simulink model "DYN_01x"  (R2018b)
(part 6 of 13)

a2*de1*m6*x6*cos(e2)^2*cos(e3)*cos(e6)*sin(e4) - a3*de1*m6*x6*cos(e2)^2*cos(e4)*cos(e5)*sin(e6) - a3*de1*m6*x6*cos(e3)^2*cos(e4)*cos(e5)*sin(e6) + 2*I6xy*de1*cos(e2)*cos(e3)*cos(e4)^2*cos(e5)^2*sin(e2)*sin(e3) - 4*I6xy*de1*cos(e2)*cos(e3)*cos(e4)^2*cos(e6)^2*sin(e2)*sin(e3) - 4*I6xy*de1*cos(e2)*cos(e3)*cos(e5)^2*cos(e6)^2*sin(e2)*sin(e3) - 4*I6zx*de1*cos(e2)*cos(e3)^2*cos(e4)*cos(e5)^2*sin(e2)*sin(e6) - 4*I6zx*de1*cos(e2)^2*cos(e3)*cos(e4)*cos(e5)^2*sin(e3)*sin(e6) - 2*I6zx*de1*cos(e2)^2*cos(e3)^2*cos(e4)*cos(e6)*sin(e4)*sin(e5) - a2*de1*m6*y6*cos(e2)^2*cos(e3)*sin(e4)*sin(e6) - a2*de1*m6*y6*cos(e2)^2*cos(e6)*sin(e3)*sin(e5) + 4*I6xx*de1*cos(e2)*cos(e3)^2*cos(e6)^2*sin(e2)*sin(e4)*sin(e5) + 4*I6xx*de1*cos(e2)^2*cos(e3)*cos(e6)^2*sin(e3)*sin(e4)*sin(e5) + 2*I6xy*de2*cos(e4)*cos(e5)^2*cos(e6)^2*sin(e2)*sin(e3)*sin(e4) + 2*I6xy*de3*cos(e4)*cos(e5)^2*cos(e6)^2*sin(e2)*sin(e3)*sin(e4) - 4*I6yy*de1*cos(e2)*cos(e3)^2*cos(e6)^2*sin(e2)*sin(e4)*sin(e5) - 4*I6yy*de1*cos(e2)^2*cos(e3)*cos(e6)^2*sin(e3)*sin(e4)*sin(e5) + 2*I6yz*de1*cos(e2)^2*cos(e3)^2*cos(e4)*sin(e4)*sin(e5)*sin(e6) + 2*de2*m6*x6^2*cos(e2)*cos(e3)*cos(e4)^2*cos(e5)*cos(e6)^2 + 2*de3*m6*x6^2*cos(e2)*cos(e3)*cos(e4)^2*cos(e5)*cos(e6)^2 - 2*de2*m6*y6^2*cos(e2)*cos(e3)*cos(e4)^2*cos(e5)*cos(e6)^2 - 2*de3*m6*y6^2*cos(e2)*cos(e3)*cos(e4)^2*cos(e5)*cos(e6)^2 - 2*de5*m6*x6*y6*cos(e2)*cos(e3)*cos(e6)^2*sin(e4) + de1*m6*y6*z6*cos(e2)^2*cos(e5)*cos(e6)*sin(e5) + de1*m6*y6*z6*cos(e3)^2*cos(e5)*cos(e6)*sin(e5) - de1*m6*y6*z6*cos(e4)^2*cos(e5)*cos(e6)*sin(e5) - a2*de1*m6*x6*cos(e2)^2*sin(e3)*sin(e5)*sin(e6) - 2*de1*m6*x6^2*cos(e2)^2*cos(e3)^2*cos(e4)*cos(e5)*sin(e4) - 2*de1*m6*x6^2*cos(e2)^2*cos(e4)*cos(e5)*cos(e6)^2*sin(e4) - 2*de1*m6*x6^2*cos(e3)^2*cos(e4)*cos(e5)*cos(e6)^2*sin(e4) - 2*de1*m6*x6*y6*cos(e2)^2*cos(e3)^2*cos(e4)^2*cos(e5)^2 + 4*de1*m6*x6*y6*cos(e2)^2*cos(e3)^2*cos(e4)^2*cos(e6)^2 + 4*de1*m6*x6*y6*cos(e2)^2*cos(e3)^2*cos(e5)^2*cos(e6)^2 - 2*de1*m6*x6*y6*cos(e2)^2*cos(e4)^2*cos(e5)^2*cos(e6)^2 - 2*de1*m6*x6*y6*cos(e3)^2*cos(e4)^2*cos(e5)^2*cos(e6)^2 + 2*de1*m6*y6^2*cos(e2)^2*cos(e3)^2*cos(e4)*cos(e5)*sin(e4) + 2*de1*m6*y6^2*cos(e2)^2*cos(e4)*cos(e5)*cos(e6)^2*sin(e4) + 2*de1*m6*y6^2*cos(e3)^2*cos(e4)*cos(e5)*cos(e6)^2*sin(e4) + de1*m6*x6*z6*cos(e2)^2*cos(e5)*sin(e5)*sin(e6) + de1*m6*x6*z6*cos(e3)^2*cos(e5)*sin(e5)*sin(e6) - de1*m6*x6*z6*cos(e4)^2*cos(e5)*sin(e5)*sin(e6) - 2*I6xy*de5*cos(e2)*cos(e3)*cos(e4)*cos(e5)*cos(e6)*sin(e6) - 2*de2*m6*x6^2*cos(e4)^2*cos(e5)*cos(e6)^2*sin(e2)*sin(e3) - 2*de3*m6*x6^2*cos(e4)^2*cos(e5)*cos(e6)^2*sin(e2)*sin(e3) + 2*de2*m6*y6^2*cos(e4)^2*cos(e5)*cos(e6)^2*sin(e2)*sin(e3) + 2*de3*m6*y6^2*cos(e4)^2*cos(e5)*cos(e6)^2*sin(e2)*sin(e3) + 2*de5*m6*x6*y6*cos(e6)^2*sin(e2)*sin(e3)*sin(e4) + I6xx*de2*cos(e2)*cos(e3)*cos(e4)*cos(e6)*sin(e4)*sin(e6) + I6xx*de3*cos(e2)*cos(e3)*cos(e4)*cos(e6)*sin(e4)*sin(e6) - I6yy*de2*cos(e2)*cos(e3)*cos(e4)*cos(e6)*sin(e4)*sin(e6) - I6yy*de3*cos(e2)*cos(e3)*cos(e4)*cos(e6)*sin(e4)*sin(e6) - 4*I6xx*de1*cos(e2)^2*cos(e3)^2*cos(e4)*cos(e5)*cos(e6)^2*sin(e4) + 4*I6yy*de1*cos(e2)^2*cos(e3)^2*cos(e4)*cos(e5)*cos(e6)^2*sin(e4) - 2*I6yz*de1*cos(e2)^2*cos(e3)^2*cos(e4)^2*cos(e5)*cos(e6)*sin(e5) - 4*I6xx*de1*cos(e2)*cos(e3)*cos(e6)*sin(e2)*sin(e3)*sin(e6) + 2*I6xy*de2*cos(e2)*cos(e4)*cos(e6)*sin(e3)*sin(e5)*sin(e6) + 2*I6xy*de2*cos(e3)*cos(e4)*cos(e6)*sin(e2)*sin(e5)*sin(e6) + 2*I6xy*de3*cos(e2)*cos(e4)*cos(e6)*sin(e3)*sin(e5)*sin(e6) + 2*I6xy*de3*cos(e3)*cos(e4)*cos(e6)*sin(e2)*sin(e5)*sin(e6) - 2*I6xy*de4*cos(e2)*cos(e3)*cos(e6)*sin(e4)*sin(e5)*sin(e6) + 2*I6xy*de5*cos(e4)*cos(e5)*cos(e6)*sin(e2)*sin(e3)*sin(e6) + 4*I6yy*de1*cos(e2)*cos(e3)*cos(e6)*sin(e2)*sin(e3)*sin(e6) + 2*a3*de1*m6*x6*cos(e2)^2*cos(e3)^2*cos(e6)*sin(e4) - 2*I6zx*de1*cos(e2)^2*cos(e3)^2*cos(e4)^2*cos(e5)*sin(e5)*sin(e6) - 2*d4*de1*m6*y6*cos(e2)^2*cos(e3)^2*cos(e6)*sin(e5) - I6xx*de2*cos(e4)*cos(e6)*sin(e2)*sin(e3)*sin(e4)*sin(e6) - 4*I6xy*de1*cos(e2)*cos(e6)*sin(e2)*sin(e4)*sin(e5)*sin(e6) - I6xx*de3*cos(e4)*cos(e6)*sin(e2)*sin(e3)*sin(e4)*sin(e6) - 4*I6xy*de1*cos(e3)*cos(e6)*sin(e3)*sin(e4)*sin(e5)*sin(e6) + I6yy*de2*cos(e4)*cos(e6)*sin(e2)*sin(e3)*sin(e4)*sin(e6) + I6yy*de3*cos(e4)*cos(e6)*sin(e2)*sin(e3)*sin(e4)*sin(e6) - a1*de1*m6*y6*cos(e2)*cos(e4)*cos(e5)*cos(e6)*sin(e3) - a1*de1*m6*y6*cos(e3)*cos(e4)*cos(e5)*cos(e6)*sin(e2) + a3*de4*m6*y6*cos(e2)*cos(e4)*cos(e5)*cos(e6)*sin(e3) + a3*de4*m6*y6*cos(e3)*cos(e4)*cos(e5)*cos(e6)*sin(e2) + d4*de4*m6*x6*cos(e2)*cos(e3)*cos(e4)*cos(e5)*sin(e6) + d4*de6*m6*x6*cos(e2)*cos(e3)*cos(e5)*cos(e6)*sin(e4) + I6xx*de2*cos(e2)*cos(e3)*cos(e4)*cos(e5)^2*cos(e6)*sin(e4)*sin(e6) + I6xx*de3*cos(e2)*cos(e3)*cos(e4)*cos(e5)^2*cos(e6)*sin(e4)*sin(e6) - I6yy*de2*cos(e2)*cos(e3)*cos(e4)*cos(e5)^2*cos(e6)*sin(e4)*sin(e6) - I6yy*de3*cos(e2)*cos(e3)*cos(e4)*cos(e5)^2*cos(e6)*sin(e4)*sin(e6) + d4*de1*m6*y6*cos(e2)*cos(e4)*cos(e5)*cos(e6)*sin(e2) + d4*de1*m6*y6*cos(e3)*cos(e4)*cos(e5)*cos(e6)*sin(e3) + de6*m6*y6*z6*cos(e2)*cos(e3)*cos(e4)*cos(e5)*cos(e6) - a1*de1*m6*x6*cos(e2)*cos(e4)*cos(e5)*sin(e3)*sin(e6) - a1*de1*m6*x6*cos(e3)*cos(e4)*cos(e5)*sin(e2)*sin(e6) + a3*de4*m6*x6*cos(e2)*cos(e4)*cos(e5)*sin(e3)*sin(e6) + a3*de4*m6*x6*cos(e3)*cos(e4)*cos(e5)*sin(e2)*sin(e6) + a3*de6*m6*x6*cos(e2)*cos(e5)*cos(e6)*sin(e3)*sin(e4) + a3*de6*m6*x6*cos(e3)*cos(e5)*cos(e6)*sin(e2)*sin(e4) - a2*de1*m6*y6*cos(e2)*cos(e3)*cos(e6)*sin(e2)*sin(e5) + d4*de1*m6*x6*cos(e2)*cos(e4)*cos(e5)*sin(e2)*sin(e6) + d4*de1*m6*x6*cos(e3)*cos(e4)*cos(e5)*sin(e3)*sin(e6) + 2*I6xx*de1*cos(e2)*cos(e3)*cos(e4)^2*cos(e6)*sin(e2)*sin(e3)*sin(e6) + 2*I6xx*de1*cos(e2)*cos(e3)*cos(e5)^2*cos(e6)*sin(e2)*sin(e3)*sin(e6) - 2*I6yy*de1*cos(e2)*cos(e3)*cos(e4)^2*cos(e6)*sin(e2)*sin(e3)*sin(e6) - 2*I6yy*de1*cos(e2)*cos(e3)*cos(e5)^2*cos(e6)*sin(e2)*sin(e3)*sin(e6) - d4*de4*m6*y6*cos(e4)*cos(e5)*cos(e6)*sin(e2)*sin(e3) - d4*de5*m6*y6*cos(e2)*cos(e3)*cos(e6)*sin(e4)*sin(e5) - d4*de6*m6*y6*cos(e2)*cos(e3)*cos(e5)*sin(e4)*sin(e6) - de4*m6*x6*y6*cos(e2)*cos(e3)*cos(e4)*cos(e5)*sin(e5) + 2*de2*m6*x6*y6*cos(e2)*cos(e3)*cos(e5)*cos(e6)*sin(e6) + 2*de3*m6*x6*y6*cos(e2)*cos(e3)*cos(e5)*cos(e6)*sin(e6) + de4*m6*x6*z6*cos(e2)*cos(e3)*cos(e5)*cos(e6)*sin(e4) + de6*m6*x6*z6*cos(e2)*cos(e3)*cos(e4)*cos(e5)*sin(e6) - a2*de1*m6*x6*cos(e2)*cos(e6)*sin(e2)*sin(e3)*sin(e4) - a2*de1*m6*x6*cos(e2)*cos(e3)*sin(e2)*sin(e5)*sin(e6) - a3*de5*m6*y6*cos(e2)*cos(e6)*sin(e3)*sin(e4)*sin(e5) - a3*de5*m6*y6*cos(e3)*cos(e6)*sin(e2)*sin(e4)*sin(e5) - a3*de6*m6*y6*cos(e2)*cos(e5)*sin(e3)*sin(e4)*sin(e6) - a3*de6*m6*y6*cos(e3)*cos(e5)*sin(e2)*sin(e4)*sin(e6) - d4*de4*m6*x6*cos(e4)*cos(e5)*sin(e2)*sin(e3)*sin(e6) - d4*de5*m6*x6*cos(e2)*cos(e3)*sin(e4)*sin(e5)*sin(e6) - d4*de6*m6*x6*cos(e5)*cos(e6)*sin(e2)*sin(e3)*sin(e4) + 8*I6xy*de1*cos(e2)*cos(e3)^2*cos(e6)*sin(e2)*sin(e4)*sin(e5)*sin(e6) + 8*I6xy*de1*cos(e2)^2*cos(e3)*cos(e6)*sin(e3)*sin(e4)*sin(e5)*sin(e6) - I6xx*de2*cos(e4)*cos(e5)^2*cos(e6)*sin(e2)*sin(e3)*sin(e4)*sin(e6) - I6xx*de3*cos(e4)*cos(e5)^2*cos(e6)*sin(e2)*sin(e3)*sin(e4)*sin(e6) + I6yy*de2*cos(e4)*cos(e5)^2*cos(e6)*sin(e2)*sin(e3)*sin(e4)*sin(e6) + I6yy*de3*cos(e4)*cos(e5)^2*cos(e6)*sin(e2)*sin(e3)*sin(e4)*sin(e6) - 2*de1*m6*x6*y6*cos(e2)*cos(e4)*cos(e5)*sin(e2)*sin(e5) - 2*de1*m6*x6*y6*cos(e3)*cos(e4)*cos(e5)*sin(e3)*sin(e5) - 4*de1*m6*x6*y6*cos(e4)*cos(e5)*cos(e6)*sin(e4)*sin(e6) + de1*m6*x6*z6*cos(e2)*cos(e5)*cos(e6)*sin(e2)*sin(e4) + de1*m6*x6*z6*cos(e3)*cos(e5)*cos(e6)*sin(e3)*sin(e4) - de4*m6*y6*z6*cos(e2)*cos(e3)*cos(e5)*sin(e4)*sin(e6) - de4*m6*y6*z6*cos(e2)*cos(e5)*cos(e6)*sin(e3)*sin(e5) - de4*m6*y6*z6*cos(e3)*cos(e5)*cos(e6)*sin(e2)*sin(e5) - de6*m6*y6*z6*cos(e4)*cos(e5)*cos(e6)*sin(e2)*sin(e3) - a3*de5*m6*x6*cos(e2)*sin(e3)*sin(e4)*sin(e5)*sin(e6) - a3*de5*m6*x6*cos(e3)*sin(e2)*sin(e4)*sin(e5)*sin(e6) + a2*de1*m6*y6*cos(e2)*sin(e2)*sin(e3)*sin(e4)*sin(e6) + d4*de5*m6*y6*cos(e6)*sin(e2)*sin(e3)*sin(e4)*sin(e5) + d4*de6*m6*y6*cos(e5)*sin(e2)*sin(e3)*sin(e4)*sin(e6) - de2*m6*x6*y6*cos(e2)*cos(e5)*sin(e3)*sin(e4)*sin(e5) - de2*m6*x6*y6*cos(e3)*cos(e5)*sin(e2)*sin(e4)*sin(e5) - de3*m6*x6*y6*cos(e2)*cos(e5)*sin(e3)*sin(e4)*sin(e5) - de3*m6*x6*y6*cos(e3)*cos(e5)*sin(e2)*sin(e4)*sin(e5) + de4*m6*x6*y6*cos(e4)*cos(e5)*sin(e2)*sin(e3)*sin(e5) - 2*de2*m6*x6*y6*cos(e5)*cos(e6)*sin(e2)*sin(e3)*sin(e6) - 2*de3*m6*x6*y6*cos(e5)*cos(e6)*sin(e2)*sin(e3)*sin(e6) + 2*de5*m6*x6*y6*cos(e2)*cos(e6)*sin(e3)*sin(e5)*sin(e6) + 2*de5*m6*x6*y6*cos(e3)*cos(e6)*sin(e2)*sin(e5)*sin(e6) - de4*m6*x6*z6*cos(e5)*cos(e6)*sin(e2)*sin(e3)*sin(e4) - de4*m6*x6*z6*cos(e2)*cos(e5)*sin(e3)*sin(e5)*sin(e6) - de4*m6*x6*z6*cos(e3)*cos(e5)*sin(e2)*sin(e5)*sin(e6) - de6*m6*x6*z6*cos(e4)*cos(e5)*sin(e2)*sin(e3)*sin(e6) - de1*m6*y6*z6*cos(e2)*cos(e5)*sin(e2)*sin(e4)*sin(e6) - de1*m6*y6*z6*cos(e3)*cos(e5)*sin(e3)*sin(e4)*sin(e6) + d4*de5*m6*x6*sin(e2)*sin(e3)*sin(e4)*sin(e5)*sin(e6) + 2*de1*m6*x6^2*cos(e2)^2*cos(e3)^2*cos(e4)^2*cos(e5)^2*cos(e6)*sin(e6) - 2*de1*m6*y6^2*cos(e2)^2*cos(e3)^2*cos(e4)^2*cos(e5)^2*cos(e6)*sin(e6) + de4*m6*y6*z6*cos(e5)*sin(e2)*sin(e3)*sin(e4)*sin(e6) + a2*de1*m6*y6*cos(e2)^2*cos(e3)*cos(e4)*cos(e5)*cos(e6) + a2*de1*m6*x6*cos(e2)^2*cos(e3)*cos(e4)*cos(e5)*sin(e6) - 8*I6xy*de1*cos(e2)*cos(e3)^2*cos(e4)*cos(e5)*cos(e6)^2*sin(e2)*sin(e5) - 8*I6xy*de1*cos(e2)^2*cos(e3)*cos(e4)*cos(e5)*cos(e6)^2*sin(e3)*sin(e5) - 8*I6xy*de1*cos(e2)^2*cos(e3)^2*cos(e4)*cos(e5)*cos(e6)*sin(e4)*sin(e6) + de4*m6*y6*z6*cos(e2)*cos(e3)*cos(e4)*cos(e5)^2*cos(e6) - 2*a3*de1*m6*y6*cos(e2)*cos(e3)^2*cos(e6)*sin(e2)*sin(e5) - 2*a3*de1*m6*y6*cos(e2)^2*cos(e3)*cos(e6)*sin(e3)*sin(e5) - 2*d4*de1*m6*x6*cos(e2)*cos(e3)^2*cos(e6)*sin(e2)*sin(e4) - 2*d4*de1*m6*x6*cos(e2)^2*cos(e3)*cos(e6)*sin(e3)*sin(e4) + de2*m6*x6*y6*cos(e2)*cos(e3)*cos(e4)*cos(e5)^2*sin(e4) - 2*de2*m6*x6*y6*cos(e2)*cos(e3)*cos(e4)*cos(e6)^2*sin(e4) + de3*m6*x6*y6*cos(e2)*cos(e3)*cos(e4)*cos(e5)^2*sin(e4) - 2*de3*m6*x6*y6*cos(e2)*cos(e3)*cos(e4)*cos(e6)^2*sin(e4) - de2*m6*x6*z6*cos(e2)*cos(e3)*cos(e4)^2*cos(e6)*sin(e5) - de3*m6*x6*z6*cos(e2)*cos(e3)*cos(e4)^2*cos(e6)*sin(e5) + de4*m6*x6*z6*cos(e2)*cos(e3)*cos(e4)*cos(e5)^2*sin(e6) + 2*de1*m6*y6*z6*cos(e2)*cos(e3)^2*cos(e4)*cos(e6)*sin(e2) + 2*de1*m6*y6*z6*cos(e2)^2*cos(e3)*cos(e4)*cos(e6)*sin(e3) + 2*de1*m6*y6*z6*cos(e2)*cos(e4)*cos(e5)^2*cos(e6)*sin(e2) + 2*de1*m6*y6*z6*cos(e3)*cos(e4)*cos(e5)^2*cos(e6)*sin(e3) - 2*a3*de1*m6*x6*cos(e2)*cos(e3)^2*sin(e2)*sin(e5)*sin(e6) - 2*a3*de1*m6*x6*cos(e2)^2*cos(e3)*sin(e3)*sin(e5)*sin(e6) + 2*d4*de1*m6*y6*cos(e2)*cos(e3)^2*sin(e2)*sin(e4)*sin(e6) + 2*d4*de1*m6*y6*cos(e2)^2*cos(e3)*sin(e3)*sin(e4)*sin(e6) + 2*de1*m6*x6*y6*cos(e2)*cos(e3)*cos(e4)^2*sin(e2)*sin(e3) + 2*de1*m6*x6*y6*cos(e2)*cos(e3)*cos(e5)^2*sin(e2)*sin(e3) + 8*de1*m6*x6*y6*cos(e2)*cos(e3)*cos(e6)^2*sin(e2)*sin(e3) + 2*de1*m6*x6*z6*cos(e2)*cos(e3)^2*cos(e4)*sin(e2)*sin(e6) + 2*de1*m6*x6*z6*cos(e2)^2*cos(e3)*cos(e4)*sin(e3)*sin(e6) + 2*de1*m6*x6*z6*cos(e2)*cos(e4)*cos(e5)^2*sin(e2)*sin(e6) + 2*de1*m6*x6*z6*cos(e3)*cos(e4)*cos(e5)^2*sin(e3)*sin(e6) + de1*m6*x6*z6*cos(e2)^2*cos(e4)*cos(e6)*sin(e4)*sin(e5) + de1*m6*x6*z6*cos(e3)^2*cos(e4)*cos(e6)*sin(e4)*sin(e5) + de2*m6*y6*z6*cos(e2)*cos(e3)*cos(e4)^2*sin(e5)*sin(e6) + de2*m6*y6*z6*cos(e2)*cos(e5)^2*cos(e6)*sin(e3)*sin(e4) + de2*m6*y6*z6*cos(e3)*cos(e5)^2*cos(e6)*sin(e2)*sin(e4) + de3*m6*y6*z6*cos(e2)*cos(e3)*cos(e4)^2*sin(e5)*sin(e6) + de3*m6*y6*z6*cos(e2)*cos(e5)^2*cos(e6)*sin(e3)*sin(e4) + de3*m6*y6*z6*cos(e3)*cos(e5)^2*cos(e6)*sin(e2)*sin(e4) - de4*m6*y6*z6*cos(e4)*cos(e5)^2*cos(e6)*sin(e2)*sin(e3) - de2*m6*x6*y6*cos(e4)*cos(e5)^2*sin(e2)*sin(e3)*sin(e4) + 2*de2*m6*x6*y6*cos(e4)*cos(e6)^2*sin(e2)*sin(e3)*sin(e4) - de3*m6*x6*y6*cos(e4)*cos(e5)^2*sin(e2)*sin(e3)*sin(e4) + 2*de3*m6*x6*y6*cos(e4)*cos(e6)^2*sin(e2)*sin(e3)*sin(e4) + de2*m6*x6*z6*cos(e2)*cos(e5)^2*sin(e3)*sin(e4)*sin(e6) + de2*m6*x6*z6*cos(e3)*cos(e5)^2*sin(e2)*sin(e4)*sin(e6) + de2*m6*x6*z6*cos(e4)^2*cos(e6)*sin(e2)*sin(e3)*sin(e5) + de3*m6*x6*z6*cos(e2)*cos(e5)^2*sin(e3)*sin(e4)*sin(e6) + de3*m6*x6*z6*cos(e3)*cos(e5)^2*sin(e2)*sin(e4)*sin(e6) + de3*m6*x6*z6*cos(e4)^2*cos(e6)*sin(e2)*sin(e3)*sin(e5) - de4*m6*x6*z6*cos(e4)*cos(e5)^2*sin(e2)*sin(e3)*sin(e6) - de1*m6*y6*z6*cos(e2)^2*cos(e4)*sin(e4)*sin(e5)*sin(e6) - de1*m6*y6*z6*cos(e3)^2*cos(e4)*sin(e4)*sin(e5)*sin(e6) - I6xx*de4*cos(e2)*cos(e3)*cos(e4)*cos(e5)*cos(e6)*sin(e5)*sin(e6) + I6yz*de2*cos(e2)*cos(e3)*cos(e4)*cos(e5)*cos(e6)*sin(e4)*sin(e5) + I6yz*de3*cos(e2)*cos(e3)*cos(e4)*cos(e5)*cos(e6)*sin(e4)*sin(e5) + I6yy*de4*cos(e2)*cos(e3)*cos(e4)*cos(e5)*cos(e6)*sin(e5)*sin(e6) - 4*de1*m6*x6^2*cos(e2)*cos(e3)^2*cos(e6)^2*sin(e2)*sin(e4)*sin(e5) - 4*de1*m6*x6^2*cos(e2)^2*cos(e3)*cos(e6)^2*sin(e3)*sin(e4)*sin(e5) + 4*de1*m6*y6^2*cos(e2)*cos(e3)^2*cos(e6)^2*sin(e2)*sin(e4)*sin(e5) + 4*de1*m6*y6^2*cos(e2)^2*cos(e3)*cos(e6)^2*sin(e3)*sin(e4)*sin(e5) - de2*m6*y6*z6*cos(e4)^2*sin(e2)*sin(e3)*sin(e5)*sin(e6) - de3*m6*y6*z6*cos(e4)^2*sin(e2)*sin(e3)*sin(e5)*sin(e6) + 2*a3*de1*m6*y6*cos(e2)^2*cos(e3)^2*cos(e4)*cos(e5)*cos(e6) - 2*I6xx*de1*cos(e2)*cos(e3)*cos(e4)*cos(e5)*sin(e2)*sin(e3)*sin(e4) - 2*I6xx*de1*cos(e2)*cos(e4)*cos(e5)*cos(e6)*sin(e2)*sin(e5)*sin(e6) - 2*I6xx*de1*cos(e3)*cos(e4)*cos(e5)*cos(e6)*sin(e3)*sin(e5)*sin(e6) + 2*I6yy*de1*cos(e2)*cos(e3)*cos(e4)*cos(e5)*sin(e2)*sin(e3)*sin(e4) + 2*I6yz*de1*cos(e2)*cos(e3)*cos(e5)*cos(e6)*sin(e2)*sin(e3)*sin(e5) + 2*I6yy*de1*cos(e2)*cos(e4)*cos(e5)*cos(e6)*sin(e2)*sin(e5)*sin(e6) + 2*I6yy*de1*cos(e3)*cos(e4)*cos(e5)*cos(e6)*sin(e3)*sin(e5)*sin(e6) + I6zx*de2*cos(e2)*cos(e3)*cos(e4)*cos(e5)*sin(e4)*sin(e5)*sin(e6) + I6zx*de3*cos(e2)*cos(e3)*cos(e4)*cos(e5)*sin(e4)*sin(e5)*sin(e6) + 2*a3*de1*m6*x6*cos(e2)^2*cos(e3)^2*cos(e4)*cos(e5)*sin(e6) - 4*I6xy*de1*cos(e2)*cos(e3)*cos(e4)^2*cos(e5)^2*cos(e6)^2*sin(e2)*sin(e3) - I6xx*de2*cos(e2)*cos(e5)*cos(e6)*sin(e3)*sin(e4)*sin(e5)*sin(e6) - I6xx*de2*cos(e3)*cos(e5)*cos(e6)*sin(e2)*sin(e4)*sin(e5)*sin(e6) - I6xx*de3*cos(e2)*cos(e5)*cos(e6)*sin(e3)*sin(e4)*sin(e5)*sin(e6) - I6xx*de3*cos(e3)*cos(e5)*cos(e6)*sin(e2)*sin(e4)*sin(e5)*sin(e6) + I6xx*de4*cos(e4)*cos(e5)*cos(e6)*sin(e2)*sin(e3)*sin(e5)*sin(e6) - I6yz*de2*cos(e4)*cos(e5)*cos(e6)*sin(e2)*sin(e3)*sin(e4)*sin(e5) + I6yy*de2*cos(e2)*cos(e5)*cos(e6)*sin(e3)*sin(e4)*sin(e5)*sin(e6) + I6yy*de2*cos(e3)*cos(e5)*cos(e6)*sin(e2)*sin(e4)*sin(e5)*sin(e6) - I6yz*de3*cos(e4)*cos(e5)*cos(e6)*sin(e2)*sin(e3)*sin(e4)*sin(e5) + I6yy*de3*cos(e2)*cos(e5)*cos(e6)*sin(e3)*sin(e4)*sin(e5)*sin(e6) + I6yy*de3*cos(e3)*cos(e5)*cos(e6)*sin(e2)*sin(e4)*sin(e5)*sin(e6) - I6yy*de4*cos(e4)*cos(e5)*cos(e6)*sin(e2)*sin(e3)*sin(e5)*sin(e6) + 2*I6zx*de1*cos(e2)*cos(e3)*cos(e5)*sin(e2)*sin(e3)*sin(e5)*sin(e6) - I6zx*de2*cos(e4)*cos(e5)*sin(e2)*sin(e3)*sin(e4)*sin(e5)*sin(e6) - I6zx*de3*cos(e4)*cos(e5)*sin(e2)*sin(e3)*sin(e4)*sin(e5)*sin(e6) - de2*m6*x6^2*cos(e2)*cos(e3)*cos(e4)*cos(e6)*sin(e4)*sin(e6) - de3*m6*x6^2*cos(e2)*cos(e3)*cos(e4)*cos(e6)*sin(e4)*sin(e6) + de2*m6*y6^2*cos(e2)*cos(e3)*cos(e4)*cos(e6)*sin(e4)*sin(e6) + de3*m6*y6^2*cos(e2)*cos(e3)*cos(e4)*cos(e6)*sin(e4)*sin(e6) - 2*de1*m6*y6*z6*cos(e2)^2*cos(e3)^2*cos(e5)*cos(e6)*sin(e5) + de1*m6*y6*z6*cos(e2)^2*cos(e4)^2*cos(e5)*cos(e6)*sin(e5) + de1*m6*y6*z6*cos(e3)^2*cos(e4)^2*cos(e5)*cos(e6)*sin(e5) + 4*de1*m6*x6^2*cos(e2)^2*cos(e3)^2*cos(e4)*cos(e5)*cos(e6)^2*sin(e4) + 4*de1*m6*x6*y6*cos(e2)^2*cos(e3)^2*cos(e4)^2*cos(e5)^2*cos(e6)^2 - 4*de1*m6*y6^2*cos(e2)^2*cos(e3)^2*cos(e4)*cos(e5)*cos(e6)^2*sin(e4) + 4*de1*m6*x6^2*cos(e2)*cos(e3)*cos(e6)*sin(e2)*sin(e3)*sin(e6) - 4*de1*m6*y6^2*cos(e2)*cos(e3)*cos(e6)*sin(e2)*sin(e3)*sin(e6) - 2*de1*m6*x6*z6*cos(e2)^2*cos(e3)^2*cos(e5)*sin(e5)*sin(e6) + de1*m6*x6*z6*cos(e2)^2*cos(e4)^2*cos(e5)*sin(e5)*sin(e6) + de1*m6*x6*z6*cos(e3)^2*cos(e4)^2*cos(e5)*sin(e5)*sin(e6) + d4*de4*m6*y6*cos(e2)*cos(e3)*cos(e4)*cos(e5)*cos(e6) + de2*m6*x6^2*cos(e4)*cos(e6)*sin(e2)*sin(e3)*sin(e4)*sin(e6) + de3*m6*x6^2*cos(e4)*cos(e6)*sin(e2)*sin(e3)*sin(e4)*sin(e6) - de2*m6*y6^2*cos(e4)*cos(e6)*sin(e2)*sin(e3)*sin(e4)*sin(e6) - de3*m6*y6^2*cos(e4)*cos(e6)*sin(e2)*sin(e3)*sin(e4)*sin(e6) - de2*m6*x6^2*cos(e2)*cos(e3)*cos(e4)*cos(e5)^2*cos(e6)*sin(e4)*sin(e6) - de3*m6*x6^2*cos(e2)*cos(e3)*cos(e4)*cos(e5)^2*cos(e6)*sin(e4)*sin(e6) + de2*m6*y6^2*cos(e2)*cos(e3)*cos(e4)*cos(e5)^2*cos(e6)*sin(e4)*sin(e6) + de3*m6*y6^2*cos(e2)*cos(e3)*cos(e4)*cos(e5)^2*cos(e6)*sin(e4)*sin(e6) + 2*de2*m6*x6*y6*cos(e2)*cos(e4)*cos(e6)*sin(e3)*sin(e5)*sin(e6) + 2*de2*m6*x6*y6*cos(e3)*cos(e4)*cos(e6)*sin(e2)*sin(e5)*sin(e6) + 2*de3*m6*x6*y6*cos(e2)*cos(e4)*cos(e6)*sin(e3)*sin(e5)*sin(e6) + 2*de3*m6*x6*y6*cos(e3)*cos(e4)*cos(e6)*sin(e2)*sin(e5)*sin(e6) - 2*de4*m6*x6*y6*cos(e2)*cos(e3)*cos(e6)*sin(e4)*sin(e5)*sin(e6) + 2*de5*m6*x6*y6*cos(e4)*cos(e5)*cos(e6)*sin(e2)*sin(e3)*sin(e6) - 2*de1*m6*y6*z6*cos(e2)^2*cos(e3)^2*cos(e4)^2*cos(e5)*cos(e6)*sin(e5) - 2*de1*m6*x6^2*cos(e2)*cos(e3)*cos(e4)^2*cos(e6)*sin(e2)*sin(e3)*sin(e6) - 2*de1*m6*x6^2*cos(e2)*cos(e3)*cos(e5)^2*cos(e6)*sin(e2)*sin(e3)*sin(e6) + 2*de1*m6*y6^2*cos(e2)*cos(e3)*cos(e4)^2*cos(e6)*sin(e2)*sin(e3)*sin(e6) + 2*de1*m6*y6^2*cos(e2)*cos(e3)*cos(e5)^2*cos(e6)*sin(e2)*sin(e3)*sin(e6) - 2*de1*m6*x6*z6*cos(e2)^2*cos(e3)^2*cos(e4)^2*cos(e5)*sin(e5)*sin(e6) - 4*de1*m6*x6*y6*cos(e2)*cos(e6)*sin(e2)*sin(e4)*sin(e5)*sin(e6) - 4*de1*m6*x6*y6*cos(e3)*cos(e6)*sin(e3)*sin(e4)*sin(e5)*sin(e6) + de2*m6*x6^2*cos(e4)*cos(e5)^2*cos(e6)*sin(e2)*sin(e3)*sin(e4)*sin(e6) + de3*m6*x6^2*cos(e4)*cos(e5)^2*cos(e6)*sin(e2)*sin(e3)*sin(e4)*sin(e6) - de2*m6*y6^2*cos(e4)*cos(e5)^2*cos(e6)*sin(e2)*sin(e3)*sin(e4)*sin(e6) - de3*m6*y6^2*cos(e4)*cos(e5)^2*cos(e6)*sin(e2)*sin(e3)*sin(e4)*sin(e6) + 2*de4*m6*x6*y6*cos(e6)*sin(e2)*sin(e3)*sin(e4)*sin(e5)*sin(e6) - 2*d4*de1*m6*y6*cos(e2)*cos(e3)^2*cos(e4)*cos(e5)*cos(e6)*sin(e2) - 2*d4*de1*m6*y6*cos(e2)^2*cos(e3)*cos(e4)*cos(e5)*cos(e6)*sin(e3) - 2*d4*de1*m6*x6*cos(e2)*cos(e3)^2*cos(e4)*cos(e5)*sin(e2)*sin(e6) - 2*d4*de1*m6*x6*cos(e2)^2*cos(e3)*cos(e4)*cos(e5)*sin(e3)*sin(e6) + 2*I6xx*de1*cos(e2)*cos(e3)*cos(e4)^2*cos(e5)^2*cos(e6)*sin(e2)*sin(e3)*sin(e6) - 2*I6yy*de1*cos(e2)*cos(e3)*cos(e4)^2*cos(e5)^2*cos(e6)*sin(e2)*sin(e3)*sin(e6) - 4*de2*m6*x6*y6*cos(e2)*cos(e3)*cos(e4)^2*cos(e5)*cos(e6)*sin(e6) - 4*de3*m6*x6*y6*cos(e2)*cos(e3)*cos(e4)^2*cos(e5)*cos(e6)*sin(e6) + 2*de4*m6*x6*y6*cos(e2)*cos(e3)*cos(e4)*cos(e5)*cos(e6)^2*sin(e5) + 4*de1*m6*x6*y6*cos(e2)*cos(e3)^2*cos(e4)*cos(e5)*sin(e2)*sin(e5) + 4*de1*m6*x6*y6*cos(e2)^2*cos(e3)*cos(e4)*cos(e5)*sin(e3)*sin(e5) + 4*de1*m6*x6*y6*cos(e2)*cos(e4)*cos(e5)*cos(e6)^2*sin(e2)*sin(e5) + 4*de1*m6*x6*y6*cos(e3)*cos(e4)*cos(e5)*cos(e6)^2*sin(e3)*sin(e5) + 4*de1*m6*x6*y6*cos(e2)^2*cos(e4)*cos(e5)*cos(e6)*sin(e4)*sin(e6) + 4*de1*m6*x6*y6*cos(e3)^2*cos(e4)*cos(e5)*cos(e6)*sin(e4)*sin(e6) - 2*de1*m6*x6*z6*cos(e2)*cos(e3)^2*cos(e5)*cos(e6)*sin(e2)*sin(e4) - 2*de1*m6*x6*z6*cos(e2)^2*cos(e3)*cos(e5)*cos(e6)*sin(e3)*sin(e4) + 2*de2*m6*x6*y6*cos(e2)*cos(e5)*cos(e6)^2*sin(e3)*sin(e4)*sin(e5) + 2*de2*m6*x6*y6*cos(e3)*cos(e5)*cos(e6)^2*sin(e2)*sin(e4)*sin(e5) + 4*de2*m6*x6*y6*cos(e4)^2*cos(e5)*cos(e6)*sin(e2)*sin(e3)*sin(e6) + 2*de3*m6*x6*y6*cos(e2)*cos(e5)*cos(e6)^2*sin(e3)*sin(e4)*sin(e5) + 2*de3*m6*x6*y6*cos(e3)*cos(e5)*cos(e6)^2*sin(e2)*sin(e4)*sin(e5) + 4*de3*m6*x6*y6*cos(e4)^2*cos(e5)*cos(e6)*sin(e2)*sin(e3)*sin(e6) - 2*de4*m6*x6*y6*cos(e4)*cos(e5)*cos(e6)^2*sin(e2)*sin(e3)*sin(e5) + 2*de1*m6*y6*z6*cos(e2)*cos(e3)^2*cos(e5)*sin(e2)*sin(e4)*sin(e6) + 2*de1*m6*y6*z6*cos(e2)^2*cos(e3)*cos(e5)*sin(e3)*sin(e4)*sin(e6) + 2*I6zx*de1*cos(e2)*cos(e3)*cos(e4)*cos(e6)*sin(e2)*sin(e3)*sin(e4)*sin(e5) - 2*I6yz*de1*cos(e2)*cos(e3)*cos(e4)*sin(e2)*sin(e3)*sin(e4)*sin(e5)*sin(e6) + de4*m6*x6^2*cos(e2)*cos(e3)*cos(e4)*cos(e5)*cos(e6)*sin(e5)*sin(e6) - 2*de2*m6*x6*y6*cos(e2)*cos(e3)*cos(e4)*cos(e5)^2*cos(e6)^2*sin(e4) - 2*de3*m6*x6*y6*cos(e2)*cos(e3)*cos(e4)*cos(e5)^2*cos(e6)^2*sin(e4) - de4*m6*y6^2*cos(e2)*cos(e3)*cos(e4)*cos(e5)*cos(e6)*sin(e5)*sin(e6) - 4*de1*m6*y6*z6*cos(e2)*cos(e3)^2*cos(e4)*cos(e5)^2*cos(e6)*sin(e2) - 4*de1*m6*y6*z6*cos(e2)^2*cos(e3)*cos(e4)*cos(e5)^2*cos(e6)*sin(e3) + 2*de1*m6*x6^2*cos(e2)*cos(e3)*cos(e4)*cos(e5)*sin(e2)*sin(e3)*sin(e4) + 2*de1*m6*x6^2*cos(e2)*cos(e4)*cos(e5)*cos(e6)*sin(e2)*sin(e5)*sin(e6) + 2*de1*m6*x6^2*cos(e3)*cos(e4)*cos(e5)*cos(e6)*sin(e3)*sin(e5)*sin(e6) + 2*de1*m6*x6*y6*cos(e2)*cos(e3)*cos(e4)^2*cos(e5)^2*sin(e2)*sin(e3) - 4*de1*m6*x6*y6*cos(e2)*cos(e3)*cos(e4)^2*cos(e6)^2*sin(e2)*sin(e3) - 4*de1*m6*x6*y6*cos(e2)*cos(e3)*cos(e5)^2*cos(e6)^2*sin(e2)*sin(e3) - 2*de1*m6*y6^2*cos(e2)*cos(e3)*cos(e4)*cos(e5)*sin(e2)*sin(e3)*sin(e4) - 2*de1*m6*y6^2*cos(e2)*cos(e4)*cos(e5)*cos(e6)*sin(e2)*sin(e5)*sin(e6) - 2*de1*m6*y6^2*cos(e3)*cos(e4)*cos(e5)*cos(e6)*sin(e3)*sin(e5)*sin(e6) - 4*de1*m6*x6*z6*cos(e2)*cos(e3)^2*cos(e4)*cos(e5)^2*sin(e2)*sin(e6) - 4*de1*m6*x6*z6*cos(e2)^2*cos(e3)*cos(e4)*cos(e5)^2*sin(e3)*sin(e6) - 2*de1*m6*x6*z6*cos(e2)^2*cos(e3)^2*cos(e4)*cos(e6)*sin(e4)*sin(e5) + de2*m6*x6^2*cos(e2)*cos(e5)*cos(e6)*sin(e3)*sin(e4)*sin(e5)*sin(e6) + de2*m6*x6^2*cos(e3)*cos(e5)*cos(e6)*sin(e2)*sin(e4)*sin(e5)*sin(e6) + de3*m6*x6^2*cos(e2)*cos(e5)*cos(e6)*sin(e3)*sin(e4)*sin(e5)*sin(e6) + de3*m6*x6^2*cos(e3)*cos(e5)*cos(e6)*sin(e2)*sin(e4)*sin(e5)*sin(e6) - de4*m6*x6^2*cos(e4)*cos(e5)*cos(e6)*sin(e2)*sin(e3)*sin(e5)*sin(e6) + 2*de2*m6*x6*y6*cos(e4)*cos(e5)^2*cos(e6)^2*sin(e2)*sin(e3)*sin(e4) + 2*de3*m6*x6*y6*cos(e4)*cos(e5)^2*cos(e6)^2*sin(e2)*sin(e3)*sin(e4) - de2*m6*y6^2*cos(e2)*cos(e5)*cos(e6)*sin(e3)*sin(e4)*sin(e5)*sin(e6) - de2*m6*y6^2*cos(e3)*cos(e5)*cos(e6)*sin(e2)*sin(e4)*sin(e5)*sin(e6) - de3*m6*y6^2*cos(e2)*cos(e5)*cos(e6)*sin(e3)*sin(e4)*sin(e5)*sin(e6) - de3*m6*y6^2*cos(e3)*cos(e5)*cos(e6)*sin(e2)*sin(e4)*sin(e5)*sin(e6) + de4*m6*y6^2*cos(e4)*cos(e5)*cos(e6)*sin(e2)*sin(e3)*sin(e5)*sin(e6) + 2*de1*m6*y6*z6*cos(e2)^2*cos(e3)^2*cos(e4)*sin(e4)*sin(e5)*sin(e6) - a2*de1*m6*y6*cos(e2)*cos(e4)*cos(e5)*cos(e6)*sin(e2)*sin(e3) + 4*I6xx*de1*cos(e2)*cos(e3)*cos(e4)*cos(e5)*cos(e6)^2*sin(e2)*sin(e3)*sin(e4) + 4*I6xx*de1*cos(e2)*cos(e3)^2*cos(e4)*cos(e5)*cos(e6)*sin(e2)*sin(e5)*sin(e6) + 4*I6xx*de1*cos(e2)^2*cos(e3)*cos(e4)*cos(e5)*cos(e6)*sin(e3)*sin(e5)*sin(e6) - 4*I6yy*de1*cos(e2)*cos(e3)*cos(e4)*cos(e5)*cos(e6)^2*sin(e2)*sin(e3)*sin(e4) + 2*I6yz*de1*cos(e2)*cos(e3)*cos(e4)^2*cos(e5)*cos(e6)*sin(e2)*sin(e3)*sin(e5) - 4*I6yy*de1*cos(e2)*cos(e3)^2*cos(e4)*cos(e5)*cos(e6)*sin(e2)*sin(e5)*sin(e6) - 4*I6yy*de1*cos(e2)^2*cos(e3)*cos(e4)*cos(e5)*cos(e6)*sin(e3)*sin(e5)*sin(e6) - 2*de5*m6*x6*y6*cos(e2)*cos(e3)*cos(e4)*cos(e5)*cos(e6)*sin(e6) - 2*a3*de1*m6*x6*cos(e2)*cos(e3)*cos(e6)*sin(e2)*sin(e3)*sin(e4) - a2*de1*m6*x6*cos(e2)*cos(e4)*cos(e5)*sin(e2)*sin(e3)*sin(e6) + 2*I6zx*de1*cos(e2)*cos(e3)*cos(e4)^2*cos(e5)*sin(e2)*sin(e3)*sin(e5)*sin(e6) + 2*d4*de1*m6*y6*cos(e2)*cos(e3)*cos(e6)*sin(e2)*sin(e3)*sin(e5) + 2*a3*de1*m6*y6*cos(e2)*cos(e3)*sin(e2)*sin(e3)*sin(e4)*sin(e6) + 2*d4*de1*m6*x6*cos(e2)*cos(e3)*sin(e2)*sin(e3)*sin(e5)*sin(e6) - 2*de1*m6*x6^2*cos(e2)*cos(e3)*cos(e4)^2*cos(e5)^2*cos(e6)*sin(e2)*sin(e3)*sin(e6) + 2*de1*m6*y6^2*cos(e2)*cos(e3)*cos(e4)^2*cos(e5)^2*cos(e6)*sin(e2)*sin(e3)*sin(e6) + 8*de1*m6*x6*y6*cos(e2)*cos(e3)^2*cos(e6)*sin(e2)*sin(e4)*sin(e5)*sin(e6) + 8*de1*m6*x6*y6*cos(e2)^2*cos(e3)*cos(e6)*sin(e3)*sin(e4)*sin(e5)*sin(e6) + 8*I6xy*de1*cos(e2)*cos(e3)*cos(e4)*cos(e5)*cos(e6)*sin(e2)*sin(e3)*sin(e4)*sin(e6) - 8*de1*m6*x6*y6*cos(e2)*cos(e3)^2*cos(e4)*cos(e5)*cos(e6)^2*sin(e2)*sin(e5) - 8*de1*m6*x6*y6*cos(e2)^2*cos(e3)*cos(e4)*cos(e5)*cos(e6)^2*sin(e3)*sin(e5) - 8*de1*m6*x6*y6*cos(e2)^2*cos(e3)^2*cos(e4)*cos(e5)*cos(e6)*sin(e4)*sin(e6) - 2*a3*de1*m6*y6*cos(e2)*cos(e3)*cos(e4)*cos(e5)*cos(e6)*sin(e2)*sin(e3) - 2*a3*de1*m6*x6*cos(e2)*cos(e3)*cos(e4)*cos(e5)*sin(e2)*sin(e3)*sin(e6) + de2*m6*y6*z6*cos(e2)*cos(e3)*cos(e4)*cos(e5)*cos(e6)*sin(e4)*sin(e5) + de3*m6*y6*z6*cos(e2)*cos(e3)*cos(e4)*cos(e5)*cos(e6)*sin(e4)*sin(e5) + de2*m6*x6*z6*cos(e2)*cos(e3)*cos(e4)*cos(e5)*sin(e4)*sin(e5)*sin(e6) + de3*m6*x6*z6*cos(e2)*cos(e3)*cos(e4)*cos(e5)*sin(e4)*sin(e5)*sin(e6) + 2*de1*m6*y6*z6*cos(e2)*cos(e3)*cos(e5)*cos(e6)*sin(e2)*sin(e3)*sin(e5) - 4*de1*m6*x6^2*cos(e2)*cos(e3)*cos(e4)*cos(e5)*cos(e6)^2*sin(e2)*sin(e3)*sin(e4) - 4*de1*m6*x6^2*cos(e2)*cos(e3)^2*cos(e4)*cos(e5)*cos(e6)*sin(e2)*sin(e5)*sin(e6) - 4*de1*m6*x6^2*cos(e2)^2*cos(e3)*cos(e4)*cos(e5)*cos(e6)*sin(e3)*sin(e5)*sin(e6) - 4*de1*m6*x6*y6*cos(e2)*cos(e3)*cos(e4)^2*cos(e5)^2*cos(e6)^2*sin(e2)*sin(e3) + 4*de1*m6*y6^2*cos(e2)*cos(e3)*cos(e4)*cos(e5)*cos(e6)^2*sin(e2)*sin(e3)*sin(e4) + 4*de1*m6*y6^2*cos(e2)*cos(e3)^2*cos(e4)*cos(e5)*cos(e6)*sin(e2)*sin(e5)*sin(e6) + 4*de1*m6*y6^2*cos(e2)^2*cos(e3)*cos(e4)*cos(e5)*cos(e6)*sin(e3)*sin(e5)*sin(e6) + 2*de1*m6*x6*z6*cos(e2)*cos(e3)*cos(e5)*sin(e2)*sin(e3)*sin(e5)*sin(e6) - de2*m6*y6*z6*cos(e4)*cos(e5)*cos(e6)*sin(e2)*sin(e3)*sin(e4)*sin(e5) - de3*m6*y6*z6*cos(e4)*cos(e5)*cos(e6)*sin(e2)*sin(e3)*sin(e4)*sin(e5) - de2*m6*x6*z6*cos(e4)*cos(e5)*sin(e2)*sin(e3)*sin(e4)*sin(e5)*sin(e6) - de3*m6*x6*z6*cos(e4)*cos(e5)*sin(e2)*sin(e3)*sin(e4)*sin(e5)*sin(e6) + 2*de1*m6*x6*z6*cos(e2)*cos(e3)*cos(e4)^2*cos(e5)*sin(e2)*sin(e3)*sin(e5)*sin(e6) + 2*de1*m6*x6*z6*cos(e2)*cos(e3)*cos(e4)*cos(e6)*sin(e2)*sin(e3)*sin(e4)*sin(e5) - 2*de1*m6*y6*z6*cos(e2)*cos(e3)*cos(e4)*sin(e2)*sin(e3)*sin(e4)*sin(e5)*sin(e6) + 2*de1*m6*y6*z6*cos(e2)*cos(e3)*cos(e4)^2*cos(e5)*cos(e6)*sin(e2)*sin(e3)*sin(e5) + 8*de1*m6*x6*y6*cos(e2)*cos(e3)*cos(e4)*cos(e5)*cos(e6)*sin(e2)*sin(e3)*sin(e4)*sin(e6);
